simulink model "test_IK_validation"  (Simulink 8.3)
settings: Solver=ode45  StartTime=0.0  StopTime=2  MaxStep=Step_Time  RelTol=1e-3
settings Model: Creator=saeed  LastModifiedBy=Other
settings OptimizationCC: ExpressionDepthLimit=2147483647
settings DebuggingCC: FcnCallInpInsideContextMsg=UseLocalSettings

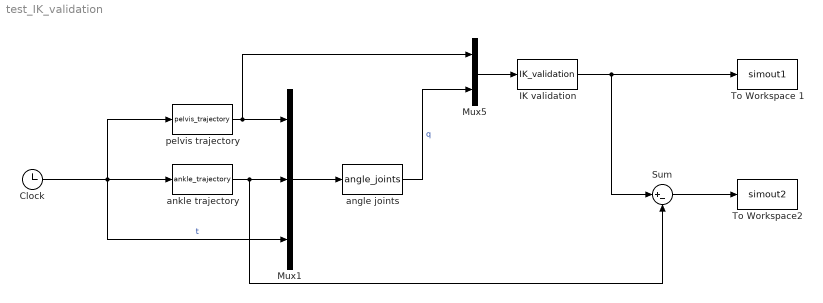
== system test_IK_validation ==
  Clock : Clock
  IK validation : MATLABFcn  MATLABFcn=IK_validation
  Mux1 : Mux  Inputs=3
  Mux5 : Mux  Inputs=2
  Sum : Sum  Inputs=|+-
  To Workspace 1 : ToWorkspace  VariableName=simout1  SaveFormat=Structure With Time  SampleTime=-1
  To Workspace2 : ToWorkspace  VariableName=simout2  SaveFormat=Structure With Time  SampleTime=-1
  angle joints : MATLABFcn  MATLABFcn=angle_joints
  ankle trajectory : MATLABFcn  MATLABFcn=ankle_trajectory
  pelvis trajectory : MATLABFcn  MATLABFcn=pelvis_trajectory
  wires:
  Clock/1 -> ankle trajectory/1, pelvis trajectory/1, Mux1/3  "t"
  IK validation/1 -> Sum/1, To Workspace 1/1
  pelvis trajectory/1 -> Mux1/1, Mux5/1
  Mux1/1 -> angle joints/1
  Mux5/1 -> IK validation/1
  angle joints/1 -> Mux5/2  "q"
  ankle trajectory/1 -> Sum/2, Mux1/2
  Sum/1 -> To Workspace2/1
